simulink model "PMSM_FOC_DbComp_2017a"  (R2023b)
settings: Solver=ode23  StartTime=0.0  StopTime=0.1  FixedStep=1e-7  MaxStep=5e-7  RelTol=1e-3
libraries: slpidlib x4, spsDCVoltageSourceLib x2, spsUniversalBridgeLib x2, spsPermanentMagnetSynchronousMachineLib x2, simulink x2, sps_lib x1
(part 1 of 2)
settings Model: Creator=Administrator  LastModifiedBy=ZJX
settings SolverCC: ZeroCrossAlgorithm=Adaptive  AlgebraicLoopSolver=TrustRegion
settings DataIOCC: ReturnWorkspaceOutputs=off
settings OptimizationCC: LifeSpan=inf
settings DebuggingCC: IgnoredZcDiagnostic=none  UnconnectedInputMsg=warning  UnconnectedOutputMsg=warning  UnconnectedLineMsg=warning  SFExecutionAtInitializationDiag=none  ArithmeticOperatorsInVariantConditions=warning
settings ModelReferenceCC: EnableRefExpFcnMdlSchedulingChecks=on
settings SFSimCC: CustomCodeUndefinedFunction=UseInterfaceOnly
settings CodeAppCC: StateflowObjectComments=on
settings SimscapeCC: SimscapeNormalizeSystem=off

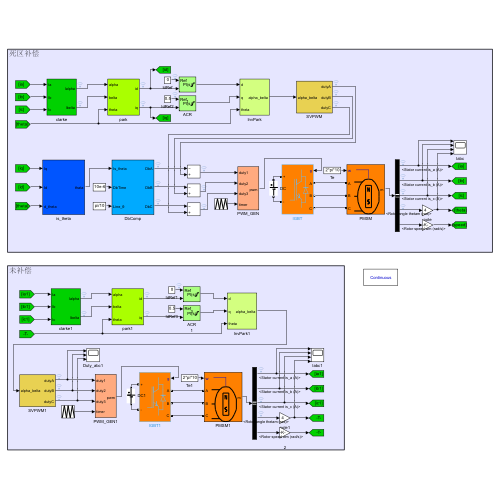
[thumbnail: Simulink's stored preview of the top-level diagram]
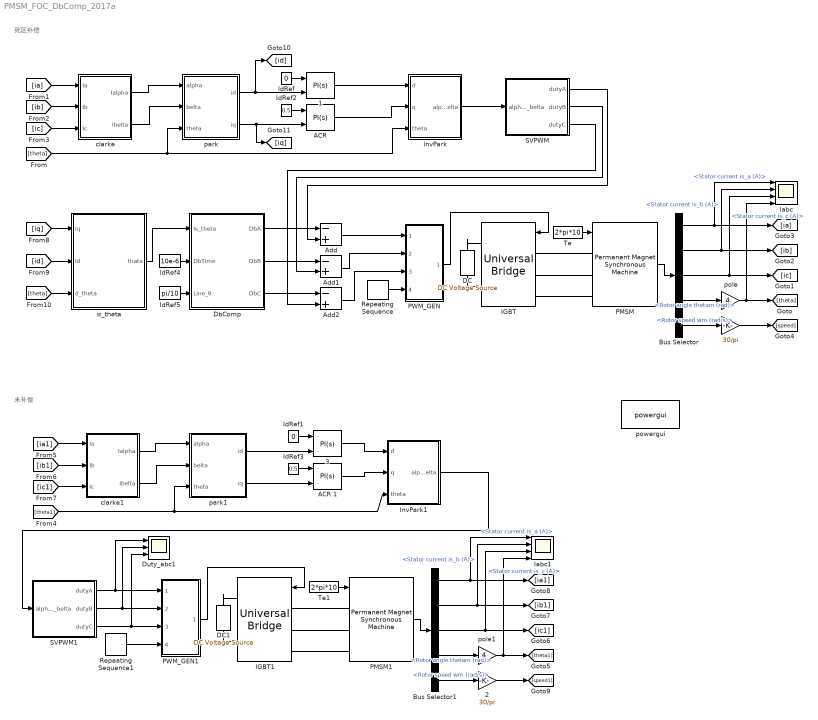
== system PMSM_FOC_DbComp_2017a ==
  note: 未补偿
  note: 死区补偿
  " " : Gain  Gain=30/pi
  " 1" : slpidlib/PID Controller (2DOF)  Controller=PI  Form=Parallel  TimeDomain=Continuous-time  UseExternalTs=off  SampleTime=-1  IntegratorMethod=Forward Euler  FilterMethod=Forward Euler  ControllerParametersSource=internal  P=10  I=300  UseKiTs=off  D=0  N=100  UseFilter=on  b=1  c=1  TunerSelectOption=Transfer Function Based (PID Tuner App)  ZeroCross=off  InitialConditionSource=internal  InitialConditionForIntegrator=0  InitialConditionForFilter=0  DifferentiatorICPrevScaledInput=0  ExternalReset=none  TrackingMode=off  Kt=1  LimitOutput=on  SatLimitsSource=internal  UpperSaturationLimit=323.3  LowerSaturationLimit=-323.3  LinearizeAsGain=on  AntiWindupMode=none  Kb=1  LimitIntegrator=off  UpperIntegratorSaturationLimit=inf  LowerIntegratorSaturationLimit=-inf  POutMin=[]  POutMax=[]  IOutMin=[]  IOutMax=[]  DOutMin=[]  DOutMax=[]  NOutMin=[]  NOutMax=[]  bOutMin=[]  bOutMax=[]  cOutMin=[]  cOutMax=[]  SumOutMin=[]  SumOutMax=[]  SaturationOutMin=[]  SaturationOutMax=[]  PParamMin=[]  PParamMax=[]  IParamMin=[]  IParamMax=[]  DParamMin=[]  DParamMax=[]  NParamMin=[]  NParamMax=[]  bParamMin=[]  bParamMax=[]  cParamMin=[]  cParamMax=[]  KbParamMin=[]  KbParamMax=[]  KtParamMin=[]  KtParamMax=[]  KbOutMin=[]  KbOutMax=[]  KtOutMin=[]  KtOutMax=[]  IntegratorOutMin=[]  IntegratorOutMax=[]  FilterOutMin=[]  FilterOutMax=[]  SumI1OutMin=[]  SumI1OutMax=[]  SumI2OutMin=[]  SumI2OutMax=[]  SumI3OutMin=[]  SumI3OutMax=[]  SumI4OutMin=[]  SumI4OutMax=[]  SumDOutMin=[]  SumDOutMax=[]  Sum1OutMin=[]  Sum1OutMax=[]  Sum2OutMin=[]  Sum2OutMax=[]  Sum3OutMin=[]  Sum3OutMax=[]  DifferentiatorOutMin=[]  DifferentiatorOutMax=[]  FilterDiffOutCoefMin=[]  FilterDiffOutCoefMax=[]  ReciprocalOutMin=[]  ReciprocalOutMax=[]  SumDenOutMin=[]  SumDenOutMax=[]  SumNumOutMin=[]  SumNumOutMax=[]  DivideOutMin=[]  DivideOutMax=[]  UdiffTsProdOutMin=[]  UdiffTsProdOutMax=[]  NTsProdOutMin=[]  NTsProdOutMax=[]  UintegralTsProdOutMin=[]  UintegralTsProdOutMax=[]  UngainTsProdOutMin=[]  UngainTsProdOutMax=[]  ClampingZeroOutDataTypeStr=Inherit: Inherit via back propagation  ClampingZeroOutMin=[]  ClampingZeroOutMax=[]  FilterDenConstantOutDataTypeStr=Inherit: Inherit via back propagation  FilterDenConstantOutMin=[]  FilterDenConstantOutMax=[]  PCopyOutDataTypeStr=Inherit: Inherit via back propagation  PCopyOutMin=[]  PCopyOutMax=[]  NCopyOutDataTypeStr=Inherit: Inherit via back propagation  NCopyOutMin=[]  NCopyOutMax=[]  IntegratorContinuousStateAttributes=''  IntegratorStateMustResolveToSignalObject=off  IntegratorRTWStateStorageClass=Auto  FilterContinuousStateAttributes=''  FilterStateMustResolveToSignalObject=off  FilterRTWStateStorageClass=Auto  ParallelPVariant=InternalParameters  IdealPVariant=Disabled  IVariant=InternalParameters  DVariant=Disabled  bVariant=InternalParameters  cVariant=Disabled  IntegratorVariant=Continuous  SatVariant=Enabled  AWVariant=Passthrough  PCopyVariant=Disabled  TRVariant=Disabled  FdbkBlocksVariant=Forward  IdealPFdbkVariant=Disabled  SatFdbkVariant=Disabled  DerivativeFilterVariant=Disabled  NVariant=Disabled  NCopyVariant=Disabled_SignalSpec  FilterICVariant=Disabled  IntegratorICVariant=InternalICs  ExternalResetVariant=Disabled  TRSumVariant=Passthrough  SumFdbkVariant=Disabled  SumVariant=Sum_PI  TsampFilterVariant=InternalTs  TsampNgainVariant=Passthrough  TsampIntegralVariant=Disabled_SignalSpec  ExternalSaturationOutDataTypeStr=Inherit: Same as second input
  " 2" : Gain  Gain=30/pi
  " 3" : slpidlib/PID Controller (2DOF)  Controller=PI  Form=Parallel  TimeDomain=Continuous-time  UseExternalTs=off  SampleTime=-1  IntegratorMethod=Forward Euler  FilterMethod=Forward Euler  ControllerParametersSource=internal  P=10  I=300  UseKiTs=off  D=0  N=100  UseFilter=on  b=1  c=1  TunerSelectOption=Transfer Function Based (PID Tuner App)  ZeroCross=off  InitialConditionSource=internal  InitialConditionForIntegrator=0  InitialConditionForFilter=0  DifferentiatorICPrevScaledInput=0  ExternalReset=none  TrackingMode=off  Kt=1  LimitOutput=on  SatLimitsSource=internal  UpperSaturationLimit=323.3  LowerSaturationLimit=-323.3  LinearizeAsGain=on  AntiWindupMode=none  Kb=1  LimitIntegrator=off  UpperIntegratorSaturationLimit=inf  LowerIntegratorSaturationLimit=-inf  POutMin=[]  POutMax=[]  IOutMin=[]  IOutMax=[]  DOutMin=[]  DOutMax=[]  NOutMin=[]  NOutMax=[]  bOutMin=[]  bOutMax=[]  cOutMin=[]  cOutMax=[]  SumOutMin=[]  SumOutMax=[]  SaturationOutMin=[]  SaturationOutMax=[]  PParamMin=[]  PParamMax=[]  IParamMin=[]  IParamMax=[]  DParamMin=[]  DParamMax=[]  NParamMin=[]  NParamMax=[]  bParamMin=[]  bParamMax=[]  cParamMin=[]  cParamMax=[]  KbParamMin=[]  KbParamMax=[]  KtParamMin=[]  KtParamMax=[]  KbOutMin=[]  KbOutMax=[]  KtOutMin=[]  KtOutMax=[]  IntegratorOutMin=[]  IntegratorOutMax=[]  FilterOutMin=[]  FilterOutMax=[]  SumI1OutMin=[]  SumI1OutMax=[]  SumI2OutMin=[]  SumI2OutMax=[]  SumI3OutMin=[]  SumI3OutMax=[]  SumI4OutMin=[]  SumI4OutMax=[]  SumDOutMin=[]  SumDOutMax=[]  Sum1OutMin=[]  Sum1OutMax=[]  Sum2OutMin=[]  Sum2OutMax=[]  Sum3OutMin=[]  Sum3OutMax=[]  DifferentiatorOutMin=[]  DifferentiatorOutMax=[]  FilterDiffOutCoefMin=[]  FilterDiffOutCoefMax=[]  ReciprocalOutMin=[]  ReciprocalOutMax=[]  SumDenOutMin=[]  SumDenOutMax=[]  SumNumOutMin=[]  SumNumOutMax=[]  DivideOutMin=[]  DivideOutMax=[]  UdiffTsProdOutMin=[]  UdiffTsProdOutMax=[]  NTsProdOutMin=[]  NTsProdOutMax=[]  UintegralTsProdOutMin=[]  UintegralTsProdOutMax=[]  UngainTsProdOutMin=[]  UngainTsProdOutMax=[]  ClampingZeroOutDataTypeStr=Inherit: Inherit via back propagation  ClampingZeroOutMin=[]  ClampingZeroOutMax=[]  FilterDenConstantOutDataTypeStr=Inherit: Inherit via back propagation  FilterDenConstantOutMin=[]  FilterDenConstantOutMax=[]  PCopyOutDataTypeStr=Inherit: Inherit via back propagation  PCopyOutMin=[]  PCopyOutMax=[]  NCopyOutDataTypeStr=Inherit: Inherit via back propagation  NCopyOutMin=[]  NCopyOutMax=[]  IntegratorContinuousStateAttributes=''  IntegratorStateMustResolveToSignalObject=off  IntegratorRTWStateStorageClass=Auto  FilterContinuousStateAttributes=''  FilterStateMustResolveToSignalObject=off  FilterRTWStateStorageClass=Auto  ParallelPVariant=InternalParameters  IdealPVariant=Disabled  IVariant=InternalParameters  DVariant=Disabled  bVariant=InternalParameters  cVariant=Disabled  IntegratorVariant=Continuous  SatVariant=Enabled  AWVariant=Passthrough  PCopyVariant=Disabled  TRVariant=Disabled  FdbkBlocksVariant=Forward  IdealPFdbkVariant=Disabled  SatFdbkVariant=Disabled  DerivativeFilterVariant=Disabled  NVariant=Disabled  NCopyVariant=Disabled_SignalSpec  FilterICVariant=Disabled  IntegratorICVariant=InternalICs  ExternalResetVariant=Disabled  TRSumVariant=Passthrough  SumFdbkVariant=Disabled  SumVariant=Sum_PI  TsampFilterVariant=InternalTs  TsampNgainVariant=Passthrough  TsampIntegralVariant=Disabled_SignalSpec  ExternalSaturationOutDataTypeStr=Inherit: Same as second input
  "ACR " : slpidlib/PID Controller (2DOF)  Controller=PI  Form=Parallel  TimeDomain=Continuous-time  UseExternalTs=off  SampleTime=-1  IntegratorMethod=Forward Euler  FilterMethod=Forward Euler  ControllerParametersSource=internal  P=10  I=300  UseKiTs=off  D=0  N=100  UseFilter=on  b=1  c=1  TunerSelectOption=Transfer Function Based (PID Tuner App)  ZeroCross=off  InitialConditionSource=internal  InitialConditionForIntegrator=0  InitialConditionForFilter=0  DifferentiatorICPrevScaledInput=0  ExternalReset=none  TrackingMode=off  Kt=1  LimitOutput=on  SatLimitsSource=internal  UpperSaturationLimit=323.3  LowerSaturationLimit=-323.3  LinearizeAsGain=on  AntiWindupMode=none  Kb=1  LimitIntegrator=off  UpperIntegratorSaturationLimit=inf  LowerIntegratorSaturationLimit=-inf  POutMin=[]  POutMax=[]  IOutMin=[]  IOutMax=[]  DOutMin=[]  DOutMax=[]  NOutMin=[]  NOutMax=[]  bOutMin=[]  bOutMax=[]  cOutMin=[]  cOutMax=[]  SumOutMin=[]  SumOutMax=[]  SaturationOutMin=[]  SaturationOutMax=[]  PParamMin=[]  PParamMax=[]  IParamMin=[]  IParamMax=[]  DParamMin=[]  DParamMax=[]  NParamMin=[]  NParamMax=[]  bParamMin=[]  bParamMax=[]  cParamMin=[]  cParamMax=[]  KbParamMin=[]  KbParamMax=[]  KtParamMin=[]  KtParamMax=[]  KbOutMin=[]  KbOutMax=[]  KtOutMin=[]  KtOutMax=[]  IntegratorOutMin=[]  IntegratorOutMax=[]  FilterOutMin=[]  FilterOutMax=[]  SumI1OutMin=[]  SumI1OutMax=[]  SumI2OutMin=[]  SumI2OutMax=[]  SumI3OutMin=[]  SumI3OutMax=[]  SumI4OutMin=[]  SumI4OutMax=[]  SumDOutMin=[]  SumDOutMax=[]  Sum1OutMin=[]  Sum1OutMax=[]  Sum2OutMin=[]  Sum2OutMax=[]  Sum3OutMin=[]  Sum3OutMax=[]  DifferentiatorOutMin=[]  DifferentiatorOutMax=[]  FilterDiffOutCoefMin=[]  FilterDiffOutCoefMax=[]  ReciprocalOutMin=[]  ReciprocalOutMax=[]  SumDenOutMin=[]  SumDenOutMax=[]  SumNumOutMin=[]  SumNumOutMax=[]  DivideOutMin=[]  DivideOutMax=[]  UdiffTsProdOutMin=[]  UdiffTsProdOutMax=[]  NTsProdOutMin=[]  NTsProdOutMax=[]  UintegralTsProdOutMin=[]  UintegralTsProdOutMax=[]  UngainTsProdOutMin=[]  UngainTsProdOutMax=[]  ClampingZeroOutDataTypeStr=Inherit: Inherit via back propagation  ClampingZeroOutMin=[]  ClampingZeroOutMax=[]  FilterDenConstantOutDataTypeStr=Inherit: Inherit via back propagation  FilterDenConstantOutMin=[]  FilterDenConstantOutMax=[]  PCopyOutDataTypeStr=Inherit: Inherit via back propagation  PCopyOutMin=[]  PCopyOutMax=[]  NCopyOutDataTypeStr=Inherit: Inherit via back propagation  NCopyOutMin=[]  NCopyOutMax=[]  IntegratorContinuousStateAttributes=''  IntegratorStateMustResolveToSignalObject=off  IntegratorRTWStateStorageClass=Auto  FilterContinuousStateAttributes=''  FilterStateMustResolveToSignalObject=off  FilterRTWStateStorageClass=Auto  ParallelPVariant=InternalParameters  IdealPVariant=Disabled  IVariant=InternalParameters  DVariant=Disabled  bVariant=InternalParameters  cVariant=Disabled  IntegratorVariant=Continuous  SatVariant=Enabled  AWVariant=Passthrough  PCopyVariant=Disabled  TRVariant=Disabled  FdbkBlocksVariant=Forward  IdealPFdbkVariant=Disabled  SatFdbkVariant=Disabled  DerivativeFilterVariant=Disabled  NVariant=Disabled  NCopyVariant=Disabled_SignalSpec  FilterICVariant=Disabled  IntegratorICVariant=InternalICs  ExternalResetVariant=Disabled  TRSumVariant=Passthrough  SumFdbkVariant=Disabled  SumVariant=Sum_PI  TsampFilterVariant=InternalTs  TsampNgainVariant=Passthrough  TsampIntegralVariant=Disabled_SignalSpec  ExternalSaturationOutDataTypeStr=Inherit: Same as second input
  ACR 1 : slpidlib/PID Controller (2DOF)  Controller=PI  Form=Parallel  TimeDomain=Continuous-time  UseExternalTs=off  SampleTime=-1  IntegratorMethod=Forward Euler  FilterMethod=Forward Euler  ControllerParametersSource=internal  P=10  I=300  UseKiTs=off  D=0  N=100  UseFilter=on  b=1  c=1  TunerSelectOption=Transfer Function Based (PID Tuner App)  ZeroCross=off  InitialConditionSource=internal  InitialConditionForIntegrator=0  InitialConditionForFilter=0  DifferentiatorICPrevScaledInput=0  ExternalReset=none  TrackingMode=off  Kt=1  LimitOutput=on  SatLimitsSource=internal  UpperSaturationLimit=323.3  LowerSaturationLimit=-323.3  LinearizeAsGain=on  AntiWindupMode=none  Kb=1  LimitIntegrator=off  UpperIntegratorSaturationLimit=inf  LowerIntegratorSaturationLimit=-inf  POutMin=[]  POutMax=[]  IOutMin=[]  IOutMax=[]  DOutMin=[]  DOutMax=[]  NOutMin=[]  NOutMax=[]  bOutMin=[]  bOutMax=[]  cOutMin=[]  cOutMax=[]  SumOutMin=[]  SumOutMax=[]  SaturationOutMin=[]  SaturationOutMax=[]  PParamMin=[]  PParamMax=[]  IParamMin=[]  IParamMax=[]  DParamMin=[]  DParamMax=[]  NParamMin=[]  NParamMax=[]  bParamMin=[]  bParamMax=[]  cParamMin=[]  cParamMax=[]  KbParamMin=[]  KbParamMax=[]  KtParamMin=[]  KtParamMax=[]  KbOutMin=[]  KbOutMax=[]  KtOutMin=[]  KtOutMax=[]  IntegratorOutMin=[]  IntegratorOutMax=[]  FilterOutMin=[]  FilterOutMax=[]  SumI1OutMin=[]  SumI1OutMax=[]  SumI2OutMin=[]  SumI2OutMax=[]  SumI3OutMin=[]  SumI3OutMax=[]  SumI4OutMin=[]  SumI4OutMax=[]  SumDOutMin=[]  SumDOutMax=[]  Sum1OutMin=[]  Sum1OutMax=[]  Sum2OutMin=[]  Sum2OutMax=[]  Sum3OutMin=[]  Sum3OutMax=[]  DifferentiatorOutMin=[]  DifferentiatorOutMax=[]  FilterDiffOutCoefMin=[]  FilterDiffOutCoefMax=[]  ReciprocalOutMin=[]  ReciprocalOutMax=[]  SumDenOutMin=[]  SumDenOutMax=[]  SumNumOutMin=[]  SumNumOutMax=[]  DivideOutMin=[]  DivideOutMax=[]  UdiffTsProdOutMin=[]  UdiffTsProdOutMax=[]  NTsProdOutMin=[]  NTsProdOutMax=[]  UintegralTsProdOutMin=[]  UintegralTsProdOutMax=[]  UngainTsProdOutMin=[]  UngainTsProdOutMax=[]  ClampingZeroOutDataTypeStr=Inherit: Inherit via back propagation  ClampingZeroOutMin=[]  ClampingZeroOutMax=[]  FilterDenConstantOutDataTypeStr=Inherit: Inherit via back propagation  FilterDenConstantOutMin=[]  FilterDenConstantOutMax=[]  PCopyOutDataTypeStr=Inherit: Inherit via back propagation  PCopyOutMin=[]  PCopyOutMax=[]  NCopyOutDataTypeStr=Inherit: Inherit via back propagation  NCopyOutMin=[]  NCopyOutMax=[]  IntegratorContinuousStateAttributes=''  IntegratorStateMustResolveToSignalObject=off  IntegratorRTWStateStorageClass=Auto  FilterContinuousStateAttributes=''  FilterStateMustResolveToSignalObject=off  FilterRTWStateStorageClass=Auto  ParallelPVariant=InternalParameters  IdealPVariant=Disabled  IVariant=InternalParameters  DVariant=Disabled  bVariant=InternalParameters  cVariant=Disabled  IntegratorVariant=Continuous  SatVariant=Enabled  AWVariant=Passthrough  PCopyVariant=Disabled  TRVariant=Disabled  FdbkBlocksVariant=Forward  IdealPFdbkVariant=Disabled  SatFdbkVariant=Disabled  DerivativeFilterVariant=Disabled  NVariant=Disabled  NCopyVariant=Disabled_SignalSpec  FilterICVariant=Disabled  IntegratorICVariant=InternalICs  ExternalResetVariant=Disabled  TRSumVariant=Passthrough  SumFdbkVariant=Disabled  SumVariant=Sum_PI  TsampFilterVariant=InternalTs  TsampNgainVariant=Passthrough  TsampIntegralVariant=Disabled_SignalSpec  ExternalSaturationOutDataTypeStr=Inherit: Same as second input
  Add : Sum  Inputs=-+
  Add1 : Sum  Inputs=-+
  Add2 : Sum  Inputs=-+
  Bus Selector : BusSelector  OutputSignals=Stator current is_a (A),Stator current is_b (A),Stator current is_c (A),Rotor angle thetam (rad),Rotor speed wm (rad/s)
  Bus Selector1 : BusSelector  OutputSignals=Stator current is_a (A),Stator current is_b (A),Stator current is_c (A),Rotor angle thetam (rad),Rotor speed wm (rad/s)
  DC : spsDCVoltageSourceLib/DC Voltage Source  Amplitude=560  Measurements=None
  DC1 : spsDCVoltageSourceLib/DC Voltage Source  Amplitude=560  Measurements=None
  DbComp : Subsystem
  Duty_abc1 : Scope  NumInputPorts=3
  IGBT : spsUniversalBridgeLib/Universal Bridge  Arms=3  SnubberResistance=1e5  SnubberCapacitance=inf  Device=IGBT / Diodes  Ron=1e-3  Lon=0  ForwardVoltages="[  0  0  ]"  ForwardVoltage=0  GTOparameters=[ 10e-6 , 20e-6 ]  IGBTparameters=[ 1e-6 , 2e-6 ]  Measurements=None  Measurements_2=None  converterType=Rectifier
  IGBT1 : spsUniversalBridgeLib/Universal Bridge  Arms=3  SnubberResistance=1e5  SnubberCapacitance=inf  Device=IGBT / Diodes  Ron=1e-3  Lon=0  ForwardVoltages="[  0  0  ]"  ForwardVoltage=0  GTOparameters=[ 10e-6 , 20e-6 ]  IGBTparameters=[ 1e-6 , 2e-6 ]  Measurements=None  Measurements_2=None  converterType=Rectifier
  Iabc : Scope  NumInputPorts=4
  Iabc1 : Scope  NumInputPorts=4
  IdRef : Constant  Value=0
  IdRef1 : Constant  Value=0
  IdRef2 : Constant  Value=0.5
  IdRef3 : Constant  Value=0.5
  IdRef4 : Constant  Value=10e-6
  IdRef5 : Constant  Value=pi/10
  InvPark : Subsystem
  InvPark1 : Subsystem
  PMSM : spsPermanentMagnetSynchronousMachineLib/Permanent Magnet Synchronous Machine  NbPhases=3  FluxDistribution=Sinusoidal  RotorType=Round  MechanicalLoad=Speed w  PresetModel="15:  87.75 Nm 560 Vdc 3000 RPM - 97.96 Nm"  ShowDetailedParameters=on  MeasurementBus=off  Resistance=0.05  Inductance=8.5e-3  dqInductances=[8.5e-3,8.5e-3]  La=0.000795  MachineConstant=Flux linkage established by magnets (V.s)  Flux=0.192  VoltageCst=139.2998  TorqueCst=1.152  Flat=120  Mechanical=[0.011 0.001417 4 0]  PolePairs=4  InitialConditions=[0,0, 0,0]  InitialConditions5ph=[0 0 0 0 0 0]  RefAngle=Aligned with phase A axis (original Park)  IterativeDiscreteModel=Trapezoidal non iterative  TsBlock=-1  TsPowergui=0
  PMSM1 : spsPermanentMagnetSynchronousMachineLib/Permanent Magnet Synchronous Machine  NbPhases=3  FluxDistribution=Sinusoidal  RotorType=Round  MechanicalLoad=Speed w  PresetModel="15:  87.75 Nm 560 Vdc 3000 RPM - 97.96 Nm"  ShowDetailedParameters=on  MeasurementBus=off  Resistance=0.05  Inductance=8.5e-3  dqInductances=[8.5e-3,8.5e-3]  La=0.000795  MachineConstant=Flux linkage established by magnets (V.s)  Flux=0.192  VoltageCst=139.2998  TorqueCst=1.152  Flat=120  Mechanical=[0.011 0.001417 4 0]  PolePairs=4  InitialConditions=[0,0, 0,0]  InitialConditions5ph=[0 0 0 0 0 0]  RefAngle=Aligned with phase A axis (original Park)  IterativeDiscreteModel=Trapezoidal non iterative  TsBlock=-1  TsPowergui=0
  PWM_GEN : Subsystem
  PWM_GEN1 : Subsystem
  Repeating Sequence : simulink/Sources/Repeating Sequence  rep_seq_t=[0 0.5e-4 1e-4]  rep_seq_y=[0 0.5e-4 0]
  Repeating Sequence1 : simulink/Sources/Repeating Sequence  rep_seq_t=[0 0.5e-4 1e-4]  rep_seq_y=[0 0.5e-4 0]
  SVPWM : Subsystem
  SVPWM1 : Subsystem
  Te : Constant  Value=2*pi*10
  Te1 : Constant  Value=2*pi*10
  clarke : Subsystem
  clarke1 : Subsystem
  is_theta : Subsystem
  park : Subsystem
  park1 : Subsystem
  pole : Gain  Gain=4
  pole1 : Gain  Gain=4
  powergui : sps_lib/powergui  Priority=1  SimulationMode=Continuous  SampleTime=1e-7  frequency=60  Iterations=50  frequencyindice=0  Pbase=100e6  ErrMax=1e-4  UnitsV=kV  UnitsW=MW  buscounter=0  FunctionMessages=off  echomessages=off  EnableUseOfTLC=off  CurrentSourceSwitches=off  DisableSnubberDevices=off  DisableRonSwitches=off  DisableVfSwitches=off  DisplayEquations=off  AutomaticDiscreteSolvers=off  SolverType=Tustin/Backward Euler (TBE)  Interpol=off  ExternalGateDelay=off  methode=off  Ts=100  x0status=blocks  SPID=off  SwTol=0  HookPort=off  NonlinearTolerance=1e-4  nMaxIteration=100  ContinueOnMaxIteration=off  RestoreLinks=warning  ResistiveCurrentMeasurement=off  Frange=[0:2:500]  Ylog=off  Xlog=on  ShowGrid=off  save=off  variable=ZData  structure=0  ZoomFFT=off  StartTime=0.0  cycles=1  DisplayStyle=1  fundamental=60  FreqAxis=off  MaxFrequency=1000  frequencyindicesteady=1  RmsSteady=1  display=off
  wires:
  Repeating Sequence/1 -> PWM_GEN/4(timer)
  PMSM/1 -> Bus Selector/1
  Te/1 -> PMSM/1
  Bus Selector/3 -> Iabc/3, [ic]  "<Stator current is_c (A)>"
  Bus Selector/2 -> Iabc/2, [ib]  "<Stator current is_b (A)>"
  Bus Selector/1 -> Iabc/1, [ia]  "<Stator current is_a (A)>"
  [theta] -> InvPark/3(theta), park/3(theta)
  clarke/1(Ialpha) -> park/1(alpha)
  Bus Selector/4 -> pole/1  "<Rotor angle thetam (rad)>"
  pole/1 -> Iabc/4, [theta]
  clarke/2(Ibelta) -> park/2(belta)
  IdRef/1 -> " 1"/1
  park/2(iq) -> [iq], "ACR "/2
  [ia] -> clarke/1(Ia)
  [ib] -> clarke/2(Ib)
  [ic] -> clarke/3(Ic)
  park/1(id) -> " 1"/2, [id]
  " 1"/1 -> InvPark/1(d)
  "ACR "/1 -> InvPark/2(q)
  InvPark/1(alpha_belta) -> SVPWM/1(alpha_belta)
  Bus Selector/5 -> " "/1  "<Rotor speed wm (rad/s)>"
  " "/1 -> [speed]
  PWM_GEN/1(pwm) -> IGBT/1
  IdRef2/1 -> "ACR "/1
  SVPWM1/1(dutyA) -> Duty_abc1/1, PWM_GEN1/1(duty1)
  SVPWM1/3(dutyC) -> PWM_GEN1/3(duty3), Duty_abc1/3
  Repeating Sequence1/1 -> PWM_GEN1/4(timer)
  PMSM1/1 -> Bus Selector1/1
  Te1/1 -> PMSM1/1
  Bus Selector1/3 -> Iabc1/3, [ic1]  "<Stator current is_c (A)>"
  Bus Selector1/2 -> Iabc1/2, [ib1]  "<Stator current is_b (A)>"
  Bus Selector1/1 -> Iabc1/1, [ia1]  "<Stator current is_a (A)>"
  [theta1] -> InvPark1/3(theta), park1/3(theta)
  clarke1/1(Ialpha) -> park1/1(alpha)
  Bus Selector1/4 -> pole1/1  "<Rotor angle thetam (rad)>"
  pole1/1 -> Iabc1/4, [theta1]
  clarke1/2(Ibelta) -> park1/2(belta)
  IdRef1/1 -> " 3"/1
  park1/2(iq) -> ACR 1/2
  [ia1] -> clarke1/1(Ia)
  [ib1] -> clarke1/2(Ib)
  [ic1] -> clarke1/3(Ic)
  park1/1(id) -> " 3"/2
  " 3"/1 -> InvPark1/1(d)
  ACR 1/1 -> InvPark1/2(q)
  InvPark1/1(alpha_belta) -> SVPWM1/1(alpha_belta)
  SVPWM1/2(dutyB) -> Duty_abc1/2, PWM_GEN1/2(duty2)
  Bus Selector1/5 -> " 2"/1  "<Rotor speed wm (rad/s)>"
  " 2"/1 -> [speed1]
  PWM_GEN1/1(pwm) -> IGBT1/1
  IdRef3/1 -> ACR 1/1
  [theta] -> is_theta/3(d_theta)
  is_theta/1(thata) -> DbComp/1(Is_theta)
  IdRef4/1 -> DbComp/2(DbTime)
  DbComp/3(DbC) -> Add2/1
  DbComp/2(DbB) -> Add1/1
  DbComp/1(DbA) -> Add/1
  SVPWM/1(dutyA) -> Add/2
  SVPWM/2(dutyB) -> Add1/2
  SVPWM/3(dutyC) -> Add2/2
  Add/1 -> PWM_GEN/1(duty1)
  Add1/1 -> PWM_GEN/2(duty2)
  Add2/1 -> PWM_GEN/3(duty3)
  [iq] -> is_theta/1(Iq)
  [id] -> is_theta/2(Id)
  IdRef5/1 -> DbComp/3(Line_θ)
  connections:
  DC/RConn1 -- IGBT/RConn1
  DC/LConn1 -- IGBT/RConn2
  PMSM/LConn1 -- IGBT/LConn1
  PMSM/LConn2 -- IGBT/LConn2
  PMSM/LConn3 -- IGBT/LConn3
  PMSM1/LConn3 -- IGBT1/LConn3
  DC1/LConn1 -- IGBT1/RConn2
  DC1/RConn1 -- IGBT1/RConn1
  PMSM1/LConn1 -- IGBT1/LConn1
  PMSM1/LConn2 -- IGBT1/LConn2

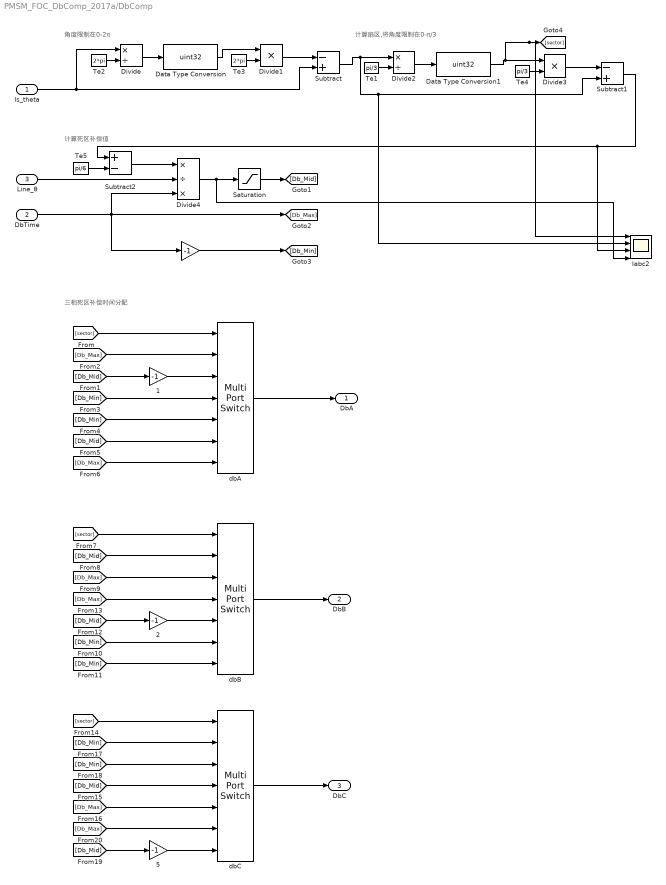
== system PMSM_FOC_DbComp_2017a/DbComp ==
  note: 三相死区补偿时间分配
  note: 计算死区补偿值
  note: 计算扇区,将角度限制在0-π/3
  note: 角度限制在0-2π
  Is_theta : Inport
  DbTime : Inport  Port=2
  Line_θ : Inport  Port=3
   {,1..2,5} (4 alike) : Gain  Gain=-1
  Data Type Conversion : DataTypeConversion  OutDataTypeStr=uint32  SaturateOnIntegerOverflow=off  RndMeth=Floor
  Data Type Conversion1 : DataTypeConversion  OutDataTypeStr=uint32  SaturateOnIntegerOverflow=off  RndMeth=Floor
  Divide : Product  Inputs=*/
  Divide1 : Product  Inputs=**
  Divide2 : Product  Inputs=*/
  Divide3 : Product  Inputs=**
  Divide4 : Product  Inputs=*/*
  Iabc2 : Scope  NumInputPorts=4
  Saturation : Saturate  UpperLimit=10e-6  LowerLimit=-10e-6
  Subtract : Sum  Inputs=-+
  Subtract1 : Sum  Inputs=-+
  Subtract2 : Sum  Inputs=+-
  Te1 : Constant  Value=pi/3
  Te2 : Constant  Value=2*pi
  Te3 : Constant  Value=2*pi
  Te4 : Constant  Value=pi/3
  Te5 : Constant  Value=pi/6
  dbA : MultiPortSwitch  DataPortOrder=Zero-based contiguous  Inputs=6  zeroidx=on  SaturateOnIntegerOverflow=off  InputSameDT=off
  dbB : MultiPortSwitch  DataPortOrder=Zero-based contiguous  Inputs=6  zeroidx=on  SaturateOnIntegerOverflow=off  InputSameDT=off
  dbC : MultiPortSwitch  DataPortOrder=Zero-based contiguous  Inputs=6  zeroidx=on  SaturateOnIntegerOverflow=off  InputSameDT=off
  DbA : Outport
  DbB : Outport  Port=2
  DbC : Outport  Port=3
  wires:
  Divide1/1 -> Subtract/1
  Data Type Conversion/1 -> Divide1/1
  Is_theta/1 -> Subtract/2, Divide/1
  Te2/1 -> Divide/2
  Divide/1 -> Data Type Conversion/1
  Te3/1 -> Divide1/2
  Te1/1 -> Divide2/2
  Divide2/1 -> Data Type Conversion1/1
  Subtract/1 -> Iabc2/2, Subtract1/2, Divide2/1
  Te4/1 -> Divide3/2
  Data Type Conversion1/1 -> [sector], Iabc2/1, Divide3/1
  Divide3/1 -> Subtract1/1
  Te5/1 -> Subtract2/2
  Subtract1/1 -> Iabc2/3, Subtract2/1
  Subtract2/1 -> Divide4/1
  Line_θ/1 -> Divide4/2
  Divide4/1 -> Iabc2/4, Saturation/1
  DbTime/1 -> " "/1, [Db_Max], Divide4/3
  " "/1 -> [Db_Min]
  [sector] -> dbA/1
  [Db_Max] -> dbA/2
  [Db_Mid] -> " 1"/1
  [Db_Min] -> dbA/5
  [Db_Mid] -> dbA/6
  [Db_Max] -> dbA/7
  [sector] -> dbB/1
  [sector] -> dbC/1
  dbC/1 -> DbC/1
  dbB/1 -> DbB/1
  dbA/1 -> DbA/1
  [Db_Max] -> dbB/3
  [Db_Max] -> dbB/4
  [Db_Mid] -> " 2"/1
  [Db_Min] -> dbB/7
  [Db_Min] -> dbC/3
  [Db_Min] -> dbC/2
  [Db_Mid] -> dbC/4
  [Db_Max] -> dbC/5
  [Db_Max] -> dbC/6
  [Db_Mid] -> " 5"/1
  " 1"/1 -> dbA/3
  [Db_Min] -> dbA/4
  [Db_Min] -> dbB/6
  " 5"/1 -> dbC/7
  [Db_Mid] -> dbB/2
  " 2"/1 -> dbB/5
  Saturation/1 -> [Db_Mid]

== system PMSM_FOC_DbComp_2017a/InvPark ==
  d : Inport
  q : Inport  Port=2
  theta : Inport  Port=3
  Mux1 : Mux  Inputs=2
  Mux6 : Mux  Inputs=3
  U_alpha : Fcn  Expr=u(1)*cos(u(3))-u(2)*sin(u(3))
  U_beta : Fcn  Expr=u(1)*sin(u(3))+u(2)*cos(u(3))
  alpha_belta : Outport
  wires:
  Mux6/1 -> U_alpha/1, U_beta/1
  U_beta/1 -> Mux1/2
  Mux1/1 -> alpha_belta/1
  U_alpha/1 -> Mux1/1
  d/1 -> Mux6/1
  theta/1 -> Mux6/3
  q/1 -> Mux6/2

== system PMSM_FOC_DbComp_2017a/InvPark1 ==
  d : Inport
  q : Inport  Port=2
  theta : Inport  Port=3
  Mux1 : Mux  Inputs=2
  Mux6 : Mux  Inputs=3
  U_alpha : Fcn  Expr=u(1)*cos(u(3))-u(2)*sin(u(3))
  U_beta : Fcn  Expr=u(1)*sin(u(3))+u(2)*cos(u(3))
  alpha_belta : Outport
  wires:
  Mux6/1 -> U_alpha/1, U_beta/1
  U_beta/1 -> Mux1/2
  Mux1/1 -> alpha_belta/1
  U_alpha/1 -> Mux1/1
  d/1 -> Mux6/1
  theta/1 -> Mux6/3
  q/1 -> Mux6/2

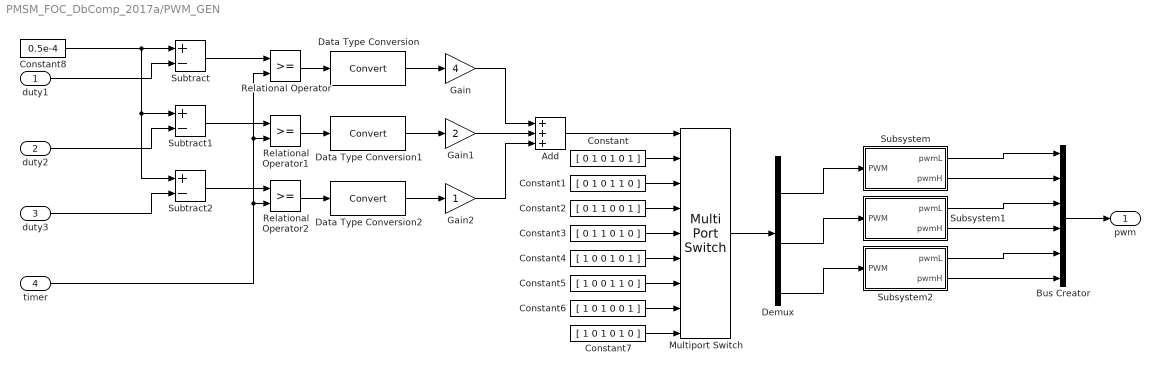
== system PMSM_FOC_DbComp_2017a/PWM_GEN ==
  duty1 : Inport
  duty2 : Inport  Port=2
  duty3 : Inport  Port=3
  timer : Inport  Port=4
  Add : Sum  Inputs=+++
  Bus Creator : BusCreator  Inputs=6
  Constant : Constant  Value=[ 0 1 0 1 0 1 ]
  Constant1 : Constant  Value=[ 0 1 0 1 1 0 ]
  Constant2 : Constant  Value=[ 0 1 1 0 0 1 ]
  Constant3 : Constant  Value=[ 0 1 1 0 1 0 ]
  Constant4 : Constant  Value=[ 1 0 0 1 0 1 ]
  Constant5 : Constant  Value=[ 1 0 0 1 1 0 ]
  Constant6 : Constant  Value=[ 1 0 1 0 0 1 ]
  Constant7 : Constant  Value=[ 1 0 1 0 1 0 ]
  Constant8 : Constant  Value=0.5e-4
  Data Type Conversion : DataTypeConversion  SaturateOnIntegerOverflow=off  RndMeth=Floor
  Data Type Conversion1 : DataTypeConversion  SaturateOnIntegerOverflow=off  RndMeth=Floor
  Data Type Conversion2 : DataTypeConversion  SaturateOnIntegerOverflow=off  RndMeth=Floor
  Demux : Demux  Outputs=6
  Gain : Gain  Gain=4
  Gain1 : Gain  Gain=2
  Gain2 : Gain
  Multiport Switch : MultiPortSwitch  DataPortOrder=Zero-based contiguous  Inputs=8  zeroidx=on  SaturateOnIntegerOverflow=off  InputSameDT=off
  Relational Operator : RelationalOperator  OutDataTypeStr=boolean  InputSameDT=off
  Relational Operator1 : RelationalOperator  OutDataTypeStr=boolean  InputSameDT=off
  Relational Operator2 : RelationalOperator  OutDataTypeStr=boolean  InputSameDT=off
  Subsystem : Subsystem
  Subsystem1 : Subsystem
  Subsystem2 : Subsystem
  Subtract : Sum  Inputs=+-
  Subtract1 : Sum  Inputs=+-
  Subtract2 : Sum  Inputs=+-
  pwm : Outport
  wires:
  Constant5/1 -> Multiport Switch/7
  Constant/1 -> Multiport Switch/2
  Gain/1 -> Add/1
  Constant2/1 -> Multiport Switch/4
  Relational Operator1/1 -> Data Type Conversion1/1
  Constant3/1 -> Multiport Switch/5
  timer/1 -> Relational Operator/2, Relational Operator1/2, Relational Operator2/2
  Relational Operator2/1 -> Data Type Conversion2/1
  Data Type Conversion2/1 -> Gain2/1
  Data Type Conversion/1 -> Gain/1
  Constant1/1 -> Multiport Switch/3
  Constant7/1 -> Multiport Switch/9
  Data Type Conversion1/1 -> Gain1/1
  Gain1/1 -> Add/2
  Gain2/1 -> Add/3
  Constant6/1 -> Multiport Switch/8
  Relational Operator/1 -> Data Type Conversion/1
  Add/1 -> Multiport Switch/1
  Constant4/1 -> Multiport Switch/6
  Constant8/1 -> Subtract/1, Subtract1/1, Subtract2/1
  Subtract/1 -> Relational Operator/1
  duty1/1 -> Subtract/2
  Subtract1/1 -> Relational Operator1/1
  duty2/1 -> Subtract1/2
  Subtract2/1 -> Relational Operator2/1
  duty3/1 -> Subtract2/2
  Subsystem2/1(pwmL) -> Bus Creator/5
  Subsystem1/1(pwmL) -> Bus Creator/3
  Subsystem1/2(pwmH) -> Bus Creator/4
  Subsystem2/2(pwmH) -> Bus Creator/6
  Subsystem/2(pwmH) -> Bus Creator/2
  Subsystem/1(pwmL) -> Bus Creator/1
  Demux/2 -> Subsystem/1(PWM)
  Demux/4 -> Subsystem1/1(PWM)
  Demux/6 -> Subsystem2/1(PWM)
  Multiport Switch/1 -> Demux/1
  Bus Creator/1 -> pwm/1

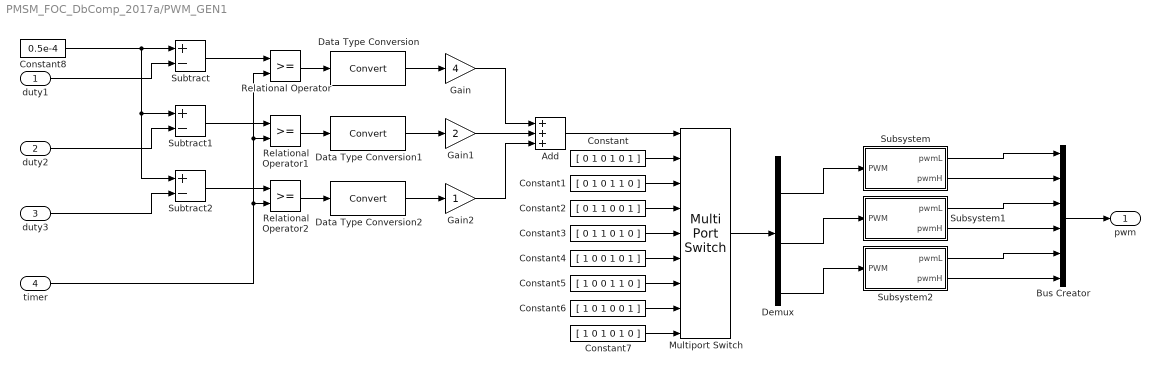
== system PMSM_FOC_DbComp_2017a/PWM_GEN1 ==
  duty1 : Inport
  duty2 : Inport  Port=2
  duty3 : Inport  Port=3
  timer : Inport  Port=4
  Add : Sum  Inputs=+++
  Bus Creator : BusCreator  Inputs=6
  Constant : Constant  Value=[ 0 1 0 1 0 1 ]
  Constant1 : Constant  Value=[ 0 1 0 1 1 0 ]
  Constant2 : Constant  Value=[ 0 1 1 0 0 1 ]
  Constant3 : Constant  Value=[ 0 1 1 0 1 0 ]
  Constant4 : Constant  Value=[ 1 0 0 1 0 1 ]
  Constant5 : Constant  Value=[ 1 0 0 1 1 0 ]
  Constant6 : Constant  Value=[ 1 0 1 0 0 1 ]
  Constant7 : Constant  Value=[ 1 0 1 0 1 0 ]
  Constant8 : Constant  Value=0.5e-4
  Data Type Conversion : DataTypeConversion  SaturateOnIntegerOverflow=off  RndMeth=Floor
  Data Type Conversion1 : DataTypeConversion  SaturateOnIntegerOverflow=off  RndMeth=Floor
  Data Type Conversion2 : DataTypeConversion  SaturateOnIntegerOverflow=off  RndMeth=Floor
  Demux : Demux  Outputs=6
  Gain : Gain  Gain=4
  Gain1 : Gain  Gain=2
  Gain2 : Gain
  Multiport Switch : MultiPortSwitch  DataPortOrder=Zero-based contiguous  Inputs=8  zeroidx=on  SaturateOnIntegerOverflow=off  InputSameDT=off
  Relational Operator : RelationalOperator  OutDataTypeStr=boolean  InputSameDT=off
  Relational Operator1 : RelationalOperator  OutDataTypeStr=boolean  InputSameDT=off
  Relational Operator2 : RelationalOperator  OutDataTypeStr=boolean  InputSameDT=off
  Subsystem : Subsystem
  Subsystem1 : Subsystem
  Subsystem2 : Subsystem
  Subtract : Sum  Inputs=+-
  Subtract1 : Sum  Inputs=+-
  Subtract2 : Sum  Inputs=+-
  pwm : Outport
  wires:
  Constant5/1 -> Multiport Switch/7
  Constant/1 -> Multiport Switch/2
  Gain/1 -> Add/1
  Constant2/1 -> Multiport Switch/4
  Relational Operator1/1 -> Data Type Conversion1/1
  Constant3/1 -> Multiport Switch/5
  timer/1 -> Relational Operator/2, Relational Operator1/2, Relational Operator2/2
  Relational Operator2/1 -> Data Type Conversion2/1
  Data Type Conversion2/1 -> Gain2/1
  Data Type Conversion/1 -> Gain/1
  Constant1/1 -> Multiport Switch/3
  Constant7/1 -> Multiport Switch/9
  Data Type Conversion1/1 -> Gain1/1
  Gain1/1 -> Add/2
  Gain2/1 -> Add/3
  Constant6/1 -> Multiport Switch/8
  Relational Operator/1 -> Data Type Conversion/1
  Add/1 -> Multiport Switch/1
  Constant4/1 -> Multiport Switch/6
  Constant8/1 -> Subtract/1, Subtract1/1, Subtract2/1
  Subtract/1 -> Relational Operator/1
  duty1/1 -> Subtract/2
  Subtract1/1 -> Relational Operator1/1
  duty2/1 -> Subtract1/2
  Subtract2/1 -> Relational Operator2/1
  duty3/1 -> Subtract2/2
  Subsystem2/1(pwmL) -> Bus Creator/5
  Subsystem1/1(pwmL) -> Bus Creator/3
  Subsystem1/2(pwmH) -> Bus Creator/4
  Subsystem2/2(pwmH) -> Bus Creator/6
  Subsystem/2(pwmH) -> Bus Creator/2
  Subsystem/1(pwmL) -> Bus Creator/1
  Demux/2 -> Subsystem/1(PWM)
  Demux/4 -> Subsystem1/1(PWM)
  Demux/6 -> Subsystem2/1(PWM)
  Multiport Switch/1 -> Demux/1
  Bus Creator/1 -> pwm/1

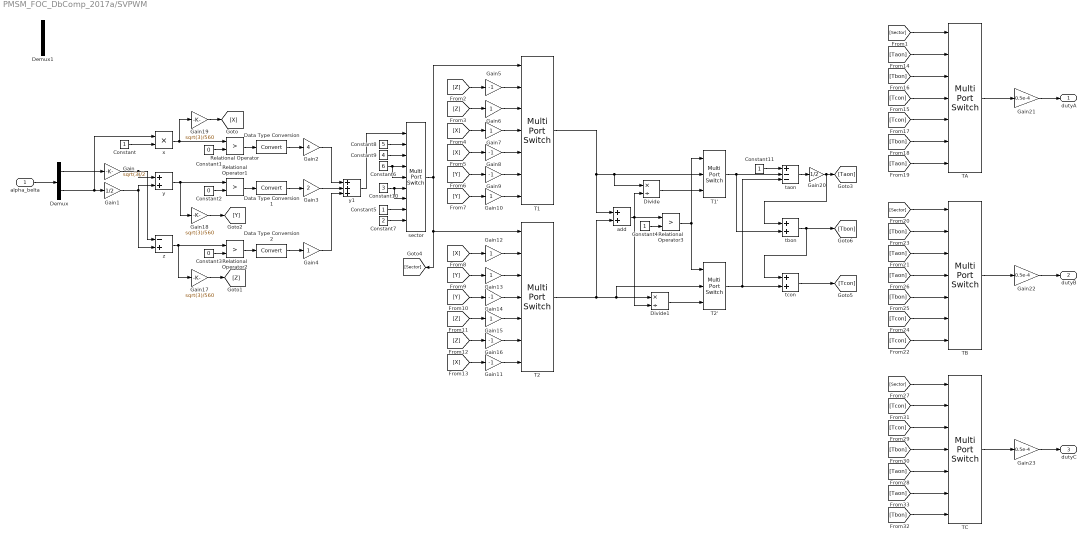
== system PMSM_FOC_DbComp_2017a/SVPWM ==
  alpha_belta : Inport
  Constant{,4..5,11} (4 alike) : Constant
  Constant1 : Constant  Value=0
  Constant10 : Constant  Value=3
  Constant2 : Constant  Value=0
  Constant3 : Constant  Value=0
  Constant6 : Constant  Value=6
  Constant7 : Constant  Value=2
  Constant8 : Constant  Value=5
  Constant9 : Constant  Value=4
  Data Type Conversion : DataTypeConversion  SaturateOnIntegerOverflow=off  RndMeth=Floor
  Data Type Conversion1 : DataTypeConversion  SaturateOnIntegerOverflow=off  RndMeth=Floor
  Data Type Conversion2 : DataTypeConversion  SaturateOnIntegerOverflow=off  RndMeth=Floor
  Demux : Demux  Outputs=2
  Demux1 : Demux  Outputs=2
  Divide : Product  Inputs=*/
  Divide1 : Product  Inputs=*/
  Gain : Gain  Gain=sqrt(3)/2
  Gain1 : Gain  Gain=1/2
  Gain{4,6..7,10,12..13,15} (7 alike) : Gain
  Gain{5,8..9,11,14,16} (6 alike) : Gain  Gain=-1
  Gain17 : Gain  Gain=sqrt(3)/560
  Gain18 : Gain  Gain=sqrt(3)/560
  Gain19 : Gain  Gain=sqrt(3)/560
  Gain2 : Gain  Gain=4
  Gain20 : Gain  Gain=1/2
  Gain21 : Gain  Gain=0.5e-4
  Gain22 : Gain  Gain=0.5e-4
  Gain23 : Gain  Gain=0.5e-4
  Gain3 : Gain  Gain=2
  Relational Operator{,1..3} (4 alike) : RelationalOperator  Operator=>  OutDataTypeStr=boolean  InputSameDT=off
  T1 : MultiPortSwitch  Inputs=6  SaturateOnIntegerOverflow=off  InputSameDT=off
  T1' : MultiPortSwitch  DataPortOrder=Zero-based contiguous  Inputs=2  zeroidx=on  SaturateOnIntegerOverflow=off  InputSameDT=off
  T2 : MultiPortSwitch  Inputs=6  SaturateOnIntegerOverflow=off  InputSameDT=off
  T2' : MultiPortSwitch  DataPortOrder=Zero-based contiguous  Inputs=2  zeroidx=on  SaturateOnIntegerOverflow=off  InputSameDT=off
  TA : MultiPortSwitch  Inputs=6  SaturateOnIntegerOverflow=off  InputSameDT=off
  TB : MultiPortSwitch  Inputs=6  SaturateOnIntegerOverflow=off  InputSameDT=off
  TC : MultiPortSwitch  Inputs=6  SaturateOnIntegerOverflow=off  InputSameDT=off
  "add " : Sum
  "sector " : MultiPortSwitch  DataPortOrder=Zero-based contiguous  Inputs=8  zeroidx=on  SaturateOnIntegerOverflow=off  InputSameDT=off
  "taon " : Sum  Inputs=+--
  tbon : Sum
  tcon : Sum
  x : Product
  y : Sum
  y1 : Sum  Inputs=+++
  z : Sum  Inputs=-+
  dutyA : Outport
  dutyB : Outport  Port=2
  dutyC : Outport  Port=3
  wires:
  [Y] -> Gain10/1
  Gain14/1 -> T2/4
  Constant10/1 -> "sector "/7, "sector "/6
  [Tcon] -> TA/5
  z/1 -> Relational Operator2/1, Gain17/1
  [Sector] -> TA/1
  Constant/1 -> x/2
  Constant9/1 -> "sector "/3
  Gain20/1 -> tbon/1, [Taon]
  Data Type Conversion/1 -> Gain2/1
  "taon "/1 -> Gain20/1
  Demux/2 -> x/1, Gain1/1
  tbon/1 -> [Tbon], tcon/1
  y1/1 -> "sector "/1
  TA/1 -> Gain21/1
  Relational Operator2/1 -> Data Type Conversion2/1
  Gain16/1 -> T2/6
  [Z] -> Gain5/1
  Constant8/1 -> "sector "/2
  Gain8/1 -> T1/5
  Gain1/1 -> y/2, z/2
  T2/1 -> T2'/2, Divide1/1, "add "/2
  [X] -> Gain11/1
  Divide1/1 -> T2'/3
  Constant6/1 -> "sector "/5, "sector "/4
  [Tbon] -> TA/3
  Constant2/1 -> Relational Operator1/2
  [Z] -> Gain15/1
  y/1 -> Gain18/1, Relational Operator1/1
  [X] -> Gain12/1
  Gain13/1 -> T2/3
  [Sector] -> TC/1
  Gain3/1 -> y1/2
  Constant4/1 -> Relational Operator3/2
  Data Type Conversion1/1 -> Gain3/1
  [Tcon] -> TC/2
  Gain4/1 -> y1/3
  Gain/1 -> y/1, z/1
  [X] -> Gain7/1
  Constant5/1 -> "sector "/8
  Data Type Conversion2/1 -> Gain4/1
  Relational Operator3/1 -> T2'/1, T1'/1
  Gain15/1 -> T2/5
  [Z] -> Gain6/1
  Gain7/1 -> T1/4
  [X] -> Gain8/1
  Gain9/1 -> T1/6
  Gain11/1 -> T2/7
  [Y] -> Gain9/1
  [Z] -> Gain16/1
  [Y] -> Gain14/1
  Gain2/1 -> y1/1
  Gain17/1 -> [Z]
  Gain18/1 -> [Y]
  Gain10/1 -> T1/7
  Divide/1 -> T1'/3
  Gain6/1 -> T1/3
  [Taon] -> TA/7
  Relational Operator/1 -> Data Type Conversion/1
  [Taon] -> TA/2
  [Tbon] -> TA/6
  Constant3/1 -> Relational Operator2/2
  [Y] -> Gain13/1
  T1'/1 -> tbon/2, "taon "/2
  [Tbon] -> TB/2
  [Taon] -> TB/3
  T1/1 -> Divide/1, T1'/2, "add "/1
  Constant7/1 -> "sector "/9
  [Tbon] -> TB/5
  [Taon] -> TB/4
  T2'/1 -> tcon/2, "taon "/3
  [Tcon] -> TB/7
  [Tcon] -> TB/6
  "add "/1 -> Divide1/2, Divide/2, Relational Operator3/1
  [Taon] -> TC/6
  [Taon] -> TC/5
  Constant1/1 -> Relational Operator/2
  tcon/1 -> [Tcon]
  Relational Operator1/1 -> Data Type Conversion1/1
  [Sector] -> TB/1
  Constant11/1 -> "taon "/1
  [Tcon] -> TC/3
  [Tcon] -> TA/4
  [Tbon] -> TC/4
  Gain5/1 -> T1/2
  x/1 -> Relational Operator/1, Gain19/1
  "sector "/1 -> [Sector], T2/1, T1/1
  Gain19/1 -> [X]
  [Tbon] -> TC/7
  Gain12/1 -> T2/2
  Gain21/1 -> dutyA/1
  Gain22/1 -> dutyB/1
  Gain23/1 -> dutyC/1
  Demux/1 -> Gain/1
  alpha_belta/1 -> Demux/1
  TB/1 -> Gain22/1
  TC/1 -> Gain23/1

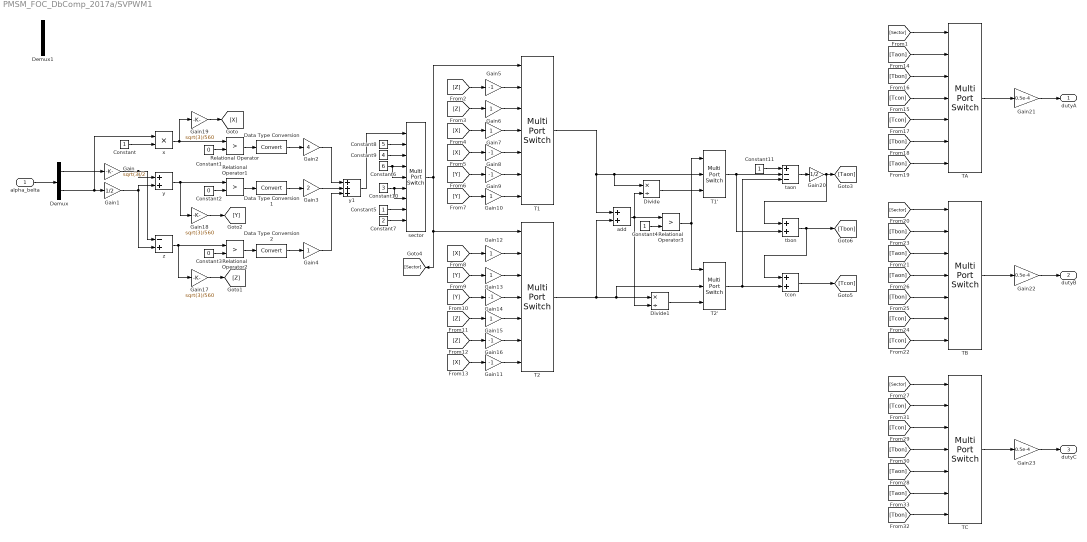
== system PMSM_FOC_DbComp_2017a/SVPWM1 ==
  alpha_belta : Inport
  Constant{,4..5,11} (4 alike) : Constant
  Constant1 : Constant  Value=0
  Constant10 : Constant  Value=3
  Constant2 : Constant  Value=0
  Constant3 : Constant  Value=0
  Constant6 : Constant  Value=6
  Constant7 : Constant  Value=2
  Constant8 : Constant  Value=5
  Constant9 : Constant  Value=4
  Data Type Conversion : DataTypeConversion  SaturateOnIntegerOverflow=off  RndMeth=Floor
  Data Type Conversion1 : DataTypeConversion  SaturateOnIntegerOverflow=off  RndMeth=Floor
  Data Type Conversion2 : DataTypeConversion  SaturateOnIntegerOverflow=off  RndMeth=Floor
  Demux : Demux  Outputs=2
  Demux1 : Demux  Outputs=2
  Divide : Product  Inputs=*/
  Divide1 : Product  Inputs=*/
  Gain : Gain  Gain=sqrt(3)/2
  Gain1 : Gain  Gain=1/2
  Gain{4,6..7,10,12..13,15} (7 alike) : Gain
  Gain{5,8..9,11,14,16} (6 alike) : Gain  Gain=-1
  Gain17 : Gain  Gain=sqrt(3)/560
  Gain18 : Gain  Gain=sqrt(3)/560
  Gain19 : Gain  Gain=sqrt(3)/560
  Gain2 : Gain  Gain=4
  Gain20 : Gain  Gain=1/2
  Gain21 : Gain  Gain=0.5e-4
  Gain22 : Gain  Gain=0.5e-4
  Gain23 : Gain  Gain=0.5e-4
  Gain3 : Gain  Gain=2
  Relational Operator{,1..3} (4 alike) : RelationalOperator  Operator=>  OutDataTypeStr=boolean  InputSameDT=off
  T1 : MultiPortSwitch  Inputs=6  SaturateOnIntegerOverflow=off  InputSameDT=off
  T1' : MultiPortSwitch  DataPortOrder=Zero-based contiguous  Inputs=2  zeroidx=on  SaturateOnIntegerOverflow=off  InputSameDT=off
  T2 : MultiPortSwitch  Inputs=6  SaturateOnIntegerOverflow=off  InputSameDT=off
  T2' : MultiPortSwitch  DataPortOrder=Zero-based contiguous  Inputs=2  zeroidx=on  SaturateOnIntegerOverflow=off  InputSameDT=off
  TA : MultiPortSwitch  Inputs=6  SaturateOnIntegerOverflow=off  InputSameDT=off
  TB : MultiPortSwitch  Inputs=6  SaturateOnIntegerOverflow=off  InputSameDT=off
  TC : MultiPortSwitch  Inputs=6  SaturateOnIntegerOverflow=off  InputSameDT=off
  "add " : Sum
  "sector " : MultiPortSwitch  DataPortOrder=Zero-based contiguous  Inputs=8  zeroidx=on  SaturateOnIntegerOverflow=off  InputSameDT=off
  "taon " : Sum  Inputs=+--
  tbon : Sum
  tcon : Sum
  x : Product
  y : Sum
  y1 : Sum  Inputs=+++
  z : Sum  Inputs=-+
  dutyA : Outport
  dutyB : Outport  Port=2
  dutyC : Outport  Port=3
  wires:
  [Y] -> Gain10/1
  Gain14/1 -> T2/4
  Constant10/1 -> "sector "/7, "sector "/6
  [Tcon] -> TA/5
  z/1 -> Relational Operator2/1, Gain17/1
  [Sector] -> TA/1
  Constant/1 -> x/2
  Constant9/1 -> "sector "/3
  Gain20/1 -> tbon/1, [Taon]
  Data Type Conversion/1 -> Gain2/1
  "taon "/1 -> Gain20/1
  Demux/2 -> x/1, Gain1/1
  tbon/1 -> [Tbon], tcon/1
  y1/1 -> "sector "/1
  TA/1 -> Gain21/1
  Relational Operator2/1 -> Data Type Conversion2/1
  Gain16/1 -> T2/6
  [Z] -> Gain5/1
  Constant8/1 -> "sector "/2
  Gain8/1 -> T1/5
  Gain1/1 -> y/2, z/2
  T2/1 -> T2'/2, Divide1/1, "add "/2
  [X] -> Gain11/1
  Divide1/1 -> T2'/3
  Constant6/1 -> "sector "/5, "sector "/4
  [Tbon] -> TA/3
  Constant2/1 -> Relational Operator1/2
  [Z] -> Gain15/1
  y/1 -> Gain18/1, Relational Operator1/1
  [X] -> Gain12/1
  Gain13/1 -> T2/3
  [Sector] -> TC/1
  Gain3/1 -> y1/2
  Constant4/1 -> Relational Operator3/2
  Data Type Conversion1/1 -> Gain3/1
  [Tcon] -> TC/2
  Gain4/1 -> y1/3
  Gain/1 -> y/1, z/1
  [X] -> Gain7/1
  Constant5/1 -> "sector "/8
  Data Type Conversion2/1 -> Gain4/1
  Relational Operator3/1 -> T2'/1, T1'/1
  Gain15/1 -> T2/5
  [Z] -> Gain6/1
  Gain7/1 -> T1/4
  [X] -> Gain8/1
  Gain9/1 -> T1/6
  Gain11/1 -> T2/7
  [Y] -> Gain9/1
  [Z] -> Gain16/1
  [Y] -> Gain14/1
  Gain2/1 -> y1/1
  Gain17/1 -> [Z]
  Gain18/1 -> [Y]
  Gain10/1 -> T1/7
  Divide/1 -> T1'/3
  Gain6/1 -> T1/3
  [Taon] -> TA/7
  Relational Operator/1 -> Data Type Conversion/1
  [Taon] -> TA/2
  [Tbon] -> TA/6
  Constant3/1 -> Relational Operator2/2
  [Y] -> Gain13/1
  T1'/1 -> tbon/2, "taon "/2
  [Tbon] -> TB/2
  [Taon] -> TB/3
  T1/1 -> Divide/1, T1'/2, "add "/1
  Constant7/1 -> "sector "/9
  [Tbon] -> TB/5
  [Taon] -> TB/4
  T2'/1 -> tcon/2, "taon "/3
  [Tcon] -> TB/7
  [Tcon] -> TB/6
  "add "/1 -> Divide1/2, Divide/2, Relational Operator3/1
  [Taon] -> TC/6
  [Taon] -> TC/5
  Constant1/1 -> Relational Operator/2
  tcon/1 -> [Tcon]
  Relational Operator1/1 -> Data Type Conversion1/1
  [Sector] -> TB/1
  Constant11/1 -> "taon "/1
  [Tcon] -> TC/3
  [Tcon] -> TA/4
  [Tbon] -> TC/4
  Gain5/1 -> T1/2
  x/1 -> Relational Operator/1, Gain19/1
  "sector "/1 -> [Sector], T2/1, T1/1
  Gain19/1 -> [X]
  [Tbon] -> TC/7
  Gain12/1 -> T2/2
  Gain21/1 -> dutyA/1
  Gain22/1 -> dutyB/1
  Gain23/1 -> dutyC/1
  Demux/1 -> Gain/1
  alpha_belta/1 -> Demux/1
  TB/1 -> Gain22/1
  TC/1 -> Gain23/1

== system PMSM_FOC_DbComp_2017a/clarke ==
  Ia : Inport
  Ib : Inport  Port=2
  Ic : Inport  Port=3
  Gain2 : Gain  Gain=2/3
  Mux : Mux  Inputs=3
  "alpha " : Fcn  Expr=u(1)-0.5*u(2)-0.5*u(3)
  belta : Fcn  Expr=sqrt(3)*0.5*u(2)-sqrt(3)*0.5*u(3)
  Ialpha : Outport
  Ibelta : Outport  Port=2
  wires:
  belta/1 -> Ibelta/1
  "alpha "/1 -> Ialpha/1
  Gain2/1 -> belta/1, "alpha "/1
  Mux/1 -> Gain2/1
  Ia/1 -> Mux/1
  Ic/1 -> Mux/3
  Ib/1 -> Mux/2

== system PMSM_FOC_DbComp_2017a/clarke1 ==
  Ia : Inport
  Ib : Inport  Port=2
  Ic : Inport  Port=3
  Gain2 : Gain  Gain=2/3
  Mux : Mux  Inputs=3
  "alpha " : Fcn  Expr=u(1)-0.5*u(2)-0.5*u(3)
  belta : Fcn  Expr=sqrt(3)*0.5*u(2)-sqrt(3)*0.5*u(3)
  Ialpha : Outport
  Ibelta : Outport  Port=2
  wires:
  belta/1 -> Ibelta/1
  "alpha "/1 -> Ialpha/1
  Gain2/1 -> belta/1, "alpha "/1
  Mux/1 -> Gain2/1
  Ia/1 -> Mux/1
  Ic/1 -> Mux/3
  Ib/1 -> Mux/2

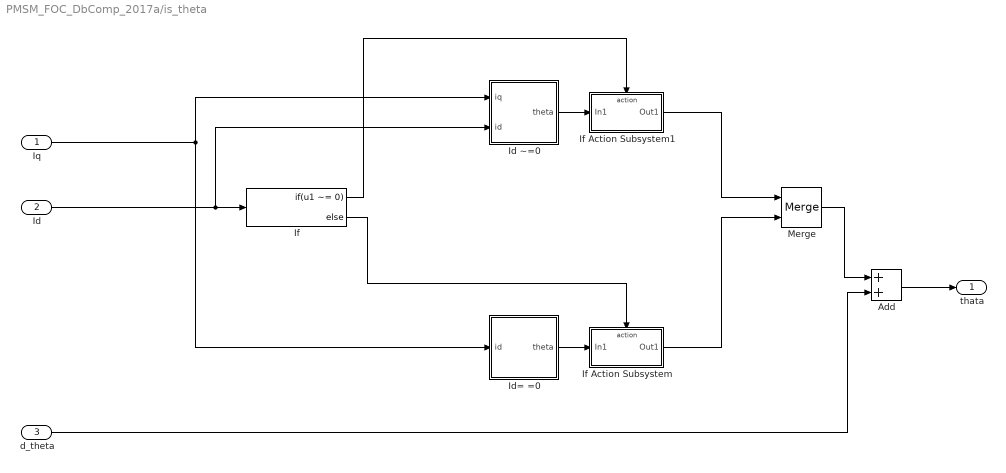
== system PMSM_FOC_DbComp_2017a/is_theta ==
  Iq : Inport
  Id : Inport  Port=2
  d_theta : Inport  Port=3
  Add : Sum
  Id ~=0 : Subsystem
  Id= =0 : Subsystem
  If : If  IfExpression=u1 ~= 0
  If Action Subsystem : Subsystem  TreatAsAtomicUnit=on
  If Action Subsystem1 : Subsystem  TreatAsAtomicUnit=on
  Merge : Merge
  thata : Outport
  wires:
  Id/1 -> Id ~=0/2(id), If/1
  If/2 -> If Action Subsystem/Action
  Iq/1 -> Id ~=0/1(iq), Id= =0/1(id)
  Id= =0/1(theta) -> If Action Subsystem/1(In1)
  If/1 -> If Action Subsystem1/Action
  Id ~=0/1(theta) -> If Action Subsystem1/1(In1)
  If Action Subsystem1/1(Out1) -> Merge/1
  If Action Subsystem/1(Out1) -> Merge/2
  Merge/1 -> Add/1
  d_theta/1 -> Add/2
  Add/1 -> thata/1

== system PMSM_FOC_DbComp_2017a/park ==
  alpha : Inport
  belta : Inport  Port=2
  theta : Inport  Port=3
  Id_fdb : Fcn  Expr=u(1)*cos(u(3))+u(2)*sin(u(3))
  Iq_fdb : Fcn  Expr=-u(1)*sin(u(3))+u(2)*cos(u(3))
  Mux4 : Mux  Inputs=3
  id : Outport
  iq : Outport  Port=2
  wires:
  Iq_fdb/1 -> iq/1
  Id_fdb/1 -> id/1
  Mux4/1 -> Id_fdb/1, Iq_fdb/1
  alpha/1 -> Mux4/1
  belta/1 -> Mux4/2
  theta/1 -> Mux4/3

== system PMSM_FOC_DbComp_2017a/park1 ==
  alpha : Inport
  belta : Inport  Port=2
  theta : Inport  Port=3
  Id_fdb : Fcn  Expr=u(1)*cos(u(3))+u(2)*sin(u(3))
  Iq_fdb : Fcn  Expr=-u(1)*sin(u(3))+u(2)*cos(u(3))
  Mux4 : Mux  Inputs=3
  id : Outport
  iq : Outport  Port=2
  wires:
  Iq_fdb/1 -> iq/1
  Id_fdb/1 -> id/1
  Mux4/1 -> Id_fdb/1, Iq_fdb/1
  alpha/1 -> Mux4/1
  belta/1 -> Mux4/2
  theta/1 -> Mux4/3

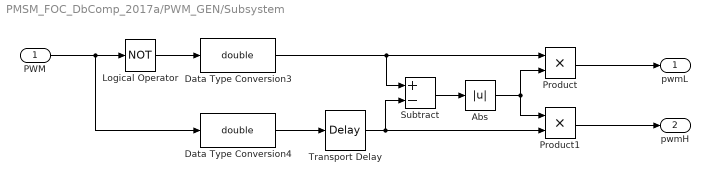
== system PMSM_FOC_DbComp_2017a/PWM_GEN/Subsystem ==
  PWM : Inport
  Abs : Abs  SaturateOnIntegerOverflow=off
  Data Type Conversion3 : DataTypeConversion  OutDataTypeStr=double  SaturateOnIntegerOverflow=off  RndMeth=Floor
  Data Type Conversion4 : DataTypeConversion  OutDataTypeStr=double  SaturateOnIntegerOverflow=off  RndMeth=Floor
  Logical Operator : Logic  Operator=NOT  AllPortsSameDT=off  OutDataTypeStr=boolean
  Product : Product
  Product1 : Product
  Subtract : Sum  Inputs=+-
  Transport Delay : TransportDelay  DelayTime=10e-6
  pwmL : Outport
  pwmH : Outport  Port=2
  wires:
  PWM/1 -> Data Type Conversion4/1, Logical Operator/1
  Subtract/1 -> Abs/1
  Transport Delay/1 -> Subtract/2, Product1/2
  Abs/1 -> Product1/1, Product/2
  Data Type Conversion3/1 -> Subtract/1, Product/1
  Product1/1 -> pwmH/1
  Product/1 -> pwmL/1
  Logical Operator/1 -> Data Type Conversion3/1
  Data Type Conversion4/1 -> Transport Delay/1

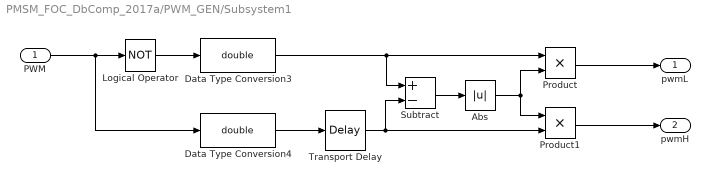
== system PMSM_FOC_DbComp_2017a/PWM_GEN/Subsystem1 ==
  PWM : Inport
  Abs : Abs  SaturateOnIntegerOverflow=off
  Data Type Conversion3 : DataTypeConversion  OutDataTypeStr=double  SaturateOnIntegerOverflow=off  RndMeth=Floor
  Data Type Conversion4 : DataTypeConversion  OutDataTypeStr=double  SaturateOnIntegerOverflow=off  RndMeth=Floor
  Logical Operator : Logic  Operator=NOT  AllPortsSameDT=off  OutDataTypeStr=boolean
  Product : Product
  Product1 : Product
  Subtract : Sum  Inputs=+-
  Transport Delay : TransportDelay  DelayTime=10e-6
  pwmL : Outport
  pwmH : Outport  Port=2
  wires:
  PWM/1 -> Data Type Conversion4/1, Logical Operator/1
  Subtract/1 -> Abs/1
  Transport Delay/1 -> Subtract/2, Product1/2
  Abs/1 -> Product1/1, Product/2
  Data Type Conversion3/1 -> Subtract/1, Product/1
  Product1/1 -> pwmH/1
  Product/1 -> pwmL/1
  Logical Operator/1 -> Data Type Conversion3/1
  Data Type Conversion4/1 -> Transport Delay/1

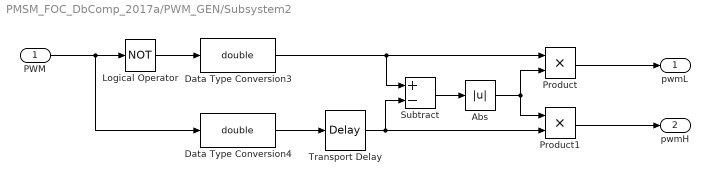
== system PMSM_FOC_DbComp_2017a/PWM_GEN/Subsystem2 ==
  PWM : Inport
  Abs : Abs  SaturateOnIntegerOverflow=off
  Data Type Conversion3 : DataTypeConversion  OutDataTypeStr=double  SaturateOnIntegerOverflow=off  RndMeth=Floor
  Data Type Conversion4 : DataTypeConversion  OutDataTypeStr=double  SaturateOnIntegerOverflow=off  RndMeth=Floor
  Logical Operator : Logic  Operator=NOT  AllPortsSameDT=off  OutDataTypeStr=boolean
  Product : Product
  Product1 : Product
  Subtract : Sum  Inputs=+-
  Transport Delay : TransportDelay  DelayTime=10e-6
  pwmL : Outport
  pwmH : Outport  Port=2
  wires:
  PWM/1 -> Data Type Conversion4/1, Logical Operator/1
  Subtract/1 -> Abs/1
  Transport Delay/1 -> Subtract/2, Product1/2
  Abs/1 -> Product1/1, Product/2
  Data Type Conversion3/1 -> Subtract/1, Product/1
  Product1/1 -> pwmH/1
  Product/1 -> pwmL/1
  Logical Operator/1 -> Data Type Conversion3/1
  Data Type Conversion4/1 -> Transport Delay/1

== system PMSM_FOC_DbComp_2017a/PWM_GEN1/Subsystem ==
  PWM : Inport
  Abs : Abs  SaturateOnIntegerOverflow=off
  Data Type Conversion3 : DataTypeConversion  OutDataTypeStr=double  SaturateOnIntegerOverflow=off  RndMeth=Floor
  Data Type Conversion4 : DataTypeConversion  OutDataTypeStr=double  SaturateOnIntegerOverflow=off  RndMeth=Floor
  Logical Operator : Logic  Operator=NOT  AllPortsSameDT=off  OutDataTypeStr=boolean
  Product : Product
  Product1 : Product
  Subtract : Sum  Inputs=+-
  Transport Delay : TransportDelay  DelayTime=10e-6
  pwmL : Outport
  pwmH : Outport  Port=2
  wires:
  PWM/1 -> Data Type Conversion4/1, Logical Operator/1
  Subtract/1 -> Abs/1
  Transport Delay/1 -> Subtract/2, Product1/2
  Abs/1 -> Product1/1, Product/2
  Data Type Conversion3/1 -> Subtract/1, Product/1
  Product1/1 -> pwmH/1
  Product/1 -> pwmL/1
  Logical Operator/1 -> Data Type Conversion3/1
  Data Type Conversion4/1 -> Transport Delay/1

== system PMSM_FOC_DbComp_2017a/PWM_GEN1/Subsystem1 ==
  PWM : Inport
  Abs : Abs  SaturateOnIntegerOverflow=off
  Data Type Conversion3 : DataTypeConversion  OutDataTypeStr=double  SaturateOnIntegerOverflow=off  RndMeth=Floor
  Data Type Conversion4 : DataTypeConversion  OutDataTypeStr=double  SaturateOnIntegerOverflow=off  RndMeth=Floor
  Logical Operator : Logic  Operator=NOT  AllPortsSameDT=off  OutDataTypeStr=boolean
  Product : Product
  Product1 : Product
  Subtract : Sum  Inputs=+-
  Transport Delay : TransportDelay  DelayTime=10e-6
  pwmL : Outport
  pwmH : Outport  Port=2
  wires:
  PWM/1 -> Data Type Conversion4/1, Logical Operator/1
  Subtract/1 -> Abs/1
  Transport Delay/1 -> Subtract/2, Product1/2
  Abs/1 -> Product1/1, Product/2
  Data Type Conversion3/1 -> Subtract/1, Product/1
  Product1/1 -> pwmH/1
  Product/1 -> pwmL/1
  Logical Operator/1 -> Data Type Conversion3/1
  Data Type Conversion4/1 -> Transport Delay/1

== system PMSM_FOC_DbComp_2017a/PWM_GEN1/Subsystem2 ==
  PWM : Inport
  Abs : Abs  SaturateOnIntegerOverflow=off
  Data Type Conversion3 : DataTypeConversion  OutDataTypeStr=double  SaturateOnIntegerOverflow=off  RndMeth=Floor
  Data Type Conversion4 : DataTypeConversion  OutDataTypeStr=double  SaturateOnIntegerOverflow=off  RndMeth=Floor
  Logical Operator : Logic  Operator=NOT  AllPortsSameDT=off  OutDataTypeStr=boolean
  Product : Product
  Product1 : Product
  Subtract : Sum  Inputs=+-
  Transport Delay : TransportDelay  DelayTime=10e-6
  pwmL : Outport
  pwmH : Outport  Port=2
  wires:
  PWM/1 -> Data Type Conversion4/1, Logical Operator/1
  Subtract/1 -> Abs/1
  Transport Delay/1 -> Subtract/2, Product1/2
  Abs/1 -> Product1/1, Product/2
  Data Type Conversion3/1 -> Subtract/1, Product/1
  Product1/1 -> pwmH/1
  Product/1 -> pwmL/1
  Logical Operator/1 -> Data Type Conversion3/1
  Data Type Conversion4/1 -> Transport Delay/1
